simulink model "sim_SMC"  (R2023a)
settings: Solver=VariableStepAuto  StartTime=0.0  StopTime=10.0  RelTol=1e-3
settings Model: Creator=Thu  LastModifiedBy=Thu

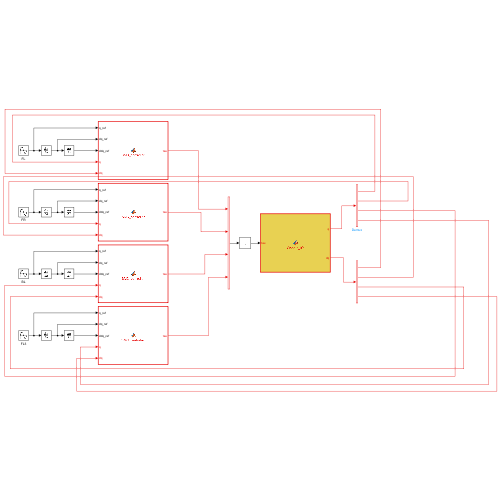
[thumbnail: Simulink's stored preview of the top-level diagram]
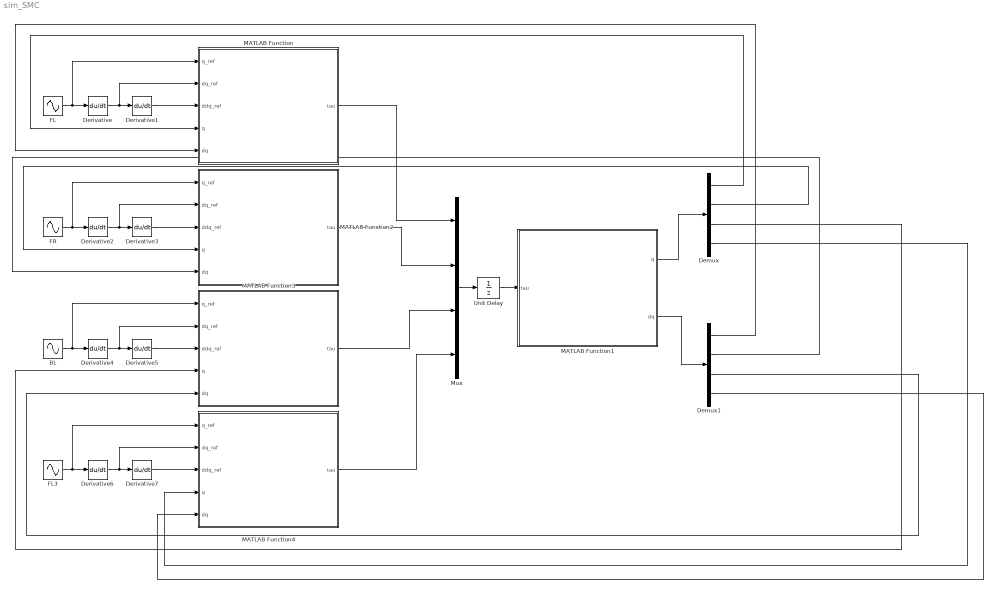
== system sim_SMC ==
  BL : Sin  Amplitude=0.2  Bias=-0.5  SampleTime=0
  Demux : Demux
  Demux1 : Demux
  Derivative{,1..7} (8 alike) : Derivative
  FL : Sin  Amplitude=0.2  Bias=-0.5  SampleTime=0
  FL3 : Sin  Amplitude=0.2  Bias=-0.5  SampleTime=0
  FR : Sin  Amplitude=0.2  Bias=-0.5  SampleTime=0
  MATLAB Function : MATLAB Function  TreatAsAtomicUnit=on
  MATLAB Function1 : MATLAB Function  TreatAsAtomicUnit=on
  MATLAB Function2 : MATLAB Function  TreatAsAtomicUnit=on
  MATLAB Function3 : MATLAB Function  TreatAsAtomicUnit=on
  MATLAB Function4 : MATLAB Function  TreatAsAtomicUnit=on
  Mux : Mux
  Unit Delay : UnitDelay  SampleTime=-1  HasFrameUpgradeWarning=on
  wires:
  FL/1 -> MATLAB Function/1(q_ref), Derivative/1
  Derivative/1 -> MATLAB Function/2(dq_ref), Derivative1/1
  Derivative1/1 -> MATLAB Function/3(ddq_ref)
  Derivative3/1 -> MATLAB Function2/3(ddq_ref)
  Derivative2/1 -> MATLAB Function2/2(dq_ref), Derivative3/1
  FR/1 -> MATLAB Function2/1(q_ref), Derivative2/1
  Derivative5/1 -> MATLAB Function3/3(ddq_ref)
  Derivative4/1 -> MATLAB Function3/2(dq_ref), Derivative5/1
  BL/1 -> MATLAB Function3/1(q_ref), Derivative4/1
  Derivative7/1 -> MATLAB Function4/3(ddq_ref)
  Derivative6/1 -> MATLAB Function4/2(dq_ref), Derivative7/1
  FL3/1 -> MATLAB Function4/1(q_ref), Derivative6/1
  MATLAB Function3/1(tau) -> Mux/3
  MATLAB Function4/1(tau) -> Mux/4
  MATLAB Function2/1(tau) -> Mux/2
  MATLAB Function/1(tau) -> Mux/1
  MATLAB Function1/1(q) -> Demux/1
  MATLAB Function1/2(dq) -> Demux1/1
  Demux/1 -> MATLAB Function/4(q)
  Demux/2 -> MATLAB Function2/4(q)
  Demux/3 -> MATLAB Function3/4(q)
  Demux/4 -> MATLAB Function4/4(q)
  Demux1/1 -> MATLAB Function/5(dq)
  Demux1/2 -> MATLAB Function2/5(dq)
  Demux1/3 -> MATLAB Function3/5(dq)
  Demux1/4 -> MATLAB Function4/5(dq)
  Mux/1 -> Unit Delay/1
  Unit Delay/1 -> MATLAB Function1/1(tau)

== matlab function sim_SMC/MATLAB Function1 ==
  data: tau input; q output; dq output
function [q, dq] = Webots_IO(tau)
    % Khai báo các hàm API từ Webots
    coder.extrinsic('wb_robot_init', 'wb_robot_step', 'wb_motor_set_torque', ...
                    'wb_position_sensor_get_value', 'wb_position_sensor_enable');    
    % Khởi tạo 8 khớp (4 chân x 2 khớp/chân)
    q = zeros(8,1);
    dq = zeros(8,1);
    persistent q_old is_initialized;
    TIME_STEP = 5; 
    
    legs = {'FL', 'FR', 'BL', 'BR'};
    parts = {'hip', 'knee'};
    
    if isempty(is_initialized)
        for i = 1:4
            for j = 1:2
                sensor_name = ['sensor_', legs{i}, '_', parts{j}];
                wb_position_sensor_enable(sensor_name, TIME_STEP);
            end
        end
        q_old = zeros(8,1);
        is_initialized = true;
    end
    
    wb_robot_step(TIME_STEP);
    
    % 2. Gửi Torque (tau) và Đọc góc (q)
    idx = 1;
    for i = 1:4
        for j = 1:2
            motor_name = ['motor_', legs{i}, '_', parts{j}];
            sensor_name = ['sensor_', legs{i}, '_', parts{j}];
            
            % Gửi lực xuống motor
            wb_motor_set_torque(motor_name, tau(idx));
            
            % Đọc góc thực tế (Radian)
            q_raw = wb_position_sensor_get_value(sensor_name);
            
            % Chuẩn hóa 0-360 độ theo logic phần cứng
            q_deg = mod(q_raw * (180/pi), 360);
            q(idx) = q_deg * (pi/180); % Đưa về Radian cho SMC
            
            idx = idx + 1;
        end
    end
    
    % 3. Tính vận tốc dq
    dt = TIME_STEP / 1000;
    dq = (q - q_old) / dt;
    q_old = q;
end

== matlab function sim_SMC/MATLAB Function ==
  data: q_ref input; tau output; dq_ref input; ddq_ref input; q input; dq input
function tau = SMC_controller(q_ref, dq_ref, ddq_ref, q, dq)
    % q_ref, dq_ref, ddq_ref: Quỹ đạo mong muốn [2x1]
    % q, dq: Phản hồi thực tế từ Webots [2x1]
    tau = zeros(2,1);
    
    %% 1. Các thông số bộ điều khiển
    lambda = [15 0; 0 15]; % Ma trận hệ số mặt trượt
    K = [5 0; 0 5];        % Độ lợi điều khiển 
    Phi = [0.1 0; 0 0.1];  % Bề dày lớp biên để chống rung 

    q1 = q(1); q2 = q(2);
    dq1 = dq(1); dq2 = dq(2);

    %% 2. Tính toán Ma trận Động lực học 
    M = [cos(q2)/50 + 0.040128, cos(q2)/100 + 0.0066948;
         cos(q2)/100 + 0.0066948, 0.0066948];
    
    C = [dq2*sin(q2)*(-0.01), sin(q2)*(dq1 + dq2)*(-0.01);
         (dq1*sin(q2))/100, 0];
    
    G = [cos(q1+q2)*0.4905 + cos(q1)*1.962;
         cos(q1+q2)*0.4905];

    %% 3. Thuật toán SMC
    e = q - q_ref;      % Sai số vị trí
    de = dq - dq_ref;   % Sai số vận tốc

    s = de + lambda * e;
    
    % điều khiển tương đương 
    tau_eq = M * (ddq_ref - lambda * de) + C * dq + G;
    
    % điều khiển bù 
    sat_s = saturation_local(s, Phi);
    
    tau_reach = -M * K * sat_s;

    %% 4. Đầu ra mô-men xoắn
    tau = tau_eq + tau_reach;
end

function out = saturation_local(s, Phi)
    out = zeros(2,1);
    for i = 1:2
        if abs(s(i)) > Phi(i,i)
            out(i) = sign(s(i));
        else
            out(i) = s(i) / Phi(i,i);
        end
    end
end

== matlab function sim_SMC/MATLAB Function2 ==
  data: q_ref input; tau output; dq_ref input; ddq_ref input; q input; dq input
function tau = SMC_controller(q_ref, dq_ref, ddq_ref, q, dq)
    % q_ref, dq_ref, ddq_ref: Quỹ đạo mong muốn [2x1]
    % q, dq: Phản hồi thực tế từ Webots [2x1]
    tau = zeros(2,1);
    
    %% 1. Các thông số bộ điều khiển
    lambda = [15 0; 0 15]; % Ma trận hệ số mặt trượt
    K = [5 0; 0 5];        % Độ lợi điều khiển 
    Phi = [0.1 0; 0 0.1];  % Bề dày lớp biên để chống rung 

    q1 = q(1); q2 = q(2);
    dq1 = dq(1); dq2 = dq(2);

    %% 2. Tính toán Ma trận Động lực học 
    M = [cos(q2)/50 + 0.040128, cos(q2)/100 + 0.0066948;
         cos(q2)/100 + 0.0066948, 0.0066948];
    
    C = [dq2*sin(q2)*(-0.01), sin(q2)*(dq1 + dq2)*(-0.01);
         (dq1*sin(q2))/100, 0];
    
    G = [cos(q1+q2)*0.4905 + cos(q1)*1.962;
         cos(q1+q2)*0.4905];

    %% 3. Thuật toán SMC
    e = q - q_ref;      % Sai số vị trí
    de = dq - dq_ref;   % Sai số vận tốc

    s = de + lambda * e;
    
    % điều khiển tương đương 
    tau_eq = M * (ddq_ref - lambda * de) + C * dq + G;
    
    % điều khiển bù 
    sat_s = saturation_local(s, Phi);
    
    tau_reach = -M * K * sat_s;

    %% 4. Đầu ra mô-men xoắn
    tau = tau_eq + tau_reach;
end

function out = saturation_local(s, Phi)
    out = zeros(2,1);
    for i = 1:2
        if abs(s(i)) > Phi(i,i)
            out(i) = sign(s(i));
        else
            out(i) = s(i) / Phi(i,i);
        end
    end
end

== matlab function sim_SMC/MATLAB Function3 ==
  data: q_ref input; tau output; dq_ref input; ddq_ref input; q input; dq input
function tau = SMC_controller(q_ref, dq_ref, ddq_ref, q, dq)
    % q_ref, dq_ref, ddq_ref: Quỹ đạo mong muốn [2x1]
    % q, dq: Phản hồi thực tế từ Webots [2x1]
    tau = zeros(2,1);
    
    %% 1. Các thông số bộ điều khiển 
    lambda = [15 0; 0 15]; % Ma trận hệ số mặt trượt
    K = [5 0; 0 5];        % Độ lợi điều khiển 
    Phi = [0.1 0; 0 0.1];  % Bề dày lớp biên để chống rung 

    q1 = q(1); q2 = q(2);
    dq1 = dq(1); dq2 = dq(2);

    %% 2. Tính toán Ma trận Động lực học 
    M = [cos(q2)/50 + 0.040128, cos(q2)/100 + 0.0066948;
         cos(q2)/100 + 0.0066948, 0.0066948];
    
    C = [dq2*sin(q2)*(-0.01), sin(q2)*(dq1 + dq2)*(-0.01);
         (dq1*sin(q2))/100, 0];
    
    G = [cos(q1+q2)*0.4905 + cos(q1)*1.962;
         cos(q1+q2)*0.4905];

    %% 3. Thuật toán SMC
    e = q - q_ref;      % Sai số vị trí
    de = dq - dq_ref;   % Sai số vận tốc

    s = de + lambda * e;
    
    % điều khiển tương đương 
    tau_eq = M * (ddq_ref - lambda * de) + C * dq + G;
    
    % điều khiển bù 
    sat_s = saturation_local(s, Phi);
    
    tau_reach = -M * K * sat_s;

    %% 4. Đầu ra mô-men xoắn
    tau = tau_eq + tau_reach;
end

function out = saturation_local(s, Phi)
    out = zeros(2,1);
    for i = 1:2
        if abs(s(i)) > Phi(i,i)
            out(i) = sign(s(i));
        else
            out(i) = s(i) / Phi(i,i);
        end
    end
end

== matlab function sim_SMC/MATLAB Function4 ==
  data: q_ref input; tau output; dq_ref input; ddq_ref input; q input; dq input
function tau = SMC_controller(q_ref, dq_ref, ddq_ref, q, dq)
    % q_ref, dq_ref, ddq_ref: Quỹ đạo mong muốn [2x1]
    % q, dq: Phản hồi thực tế từ Webots [2x1]
    tau = zeros(2,1);
    
    %% 1. Các thông số bộ điều khiển 
    lambda = [15 0; 0 15]; % Ma trận hệ số mặt trượt
    K = [5 0; 0 5];        % Độ lợi điều khiển 
    Phi = [0.1 0; 0 0.1];  % Bề dày lớp biên để chống rung 

    q1 = q(1); q2 = q(2);
    dq1 = dq(1); dq2 = dq(2);

    %% 2. Tính toán Ma trận Động lực học 
    M = [cos(q2)/50 + 0.040128, cos(q2)/100 + 0.0066948;
         cos(q2)/100 + 0.0066948, 0.0066948];
    
    C = [dq2*sin(q2)*(-0.01), sin(q2)*(dq1 + dq2)*(-0.01);
         (dq1*sin(q2))/100, 0];
    
    G = [cos(q1+q2)*0.4905 + cos(q1)*1.962;
         cos(q1+q2)*0.4905];

    %% 3. Thuật toán SMC
    e = q - q_ref;      % Sai số vị trí
    de = dq - dq_ref;   % Sai số vận tốc

    s = de + lambda * e;
    
    % điều khiển tương đương 
    tau_eq = M * (ddq_ref - lambda * de) + C * dq + G;
    
    % điều khiển bù 
    sat_s = saturation_local(s, Phi);
    
    tau_reach = -M * K * sat_s;

    %% 4. Đầu ra mô-men xoắn
    tau = tau_eq + tau_reach;
end

function out = saturation_local(s, Phi)
    out = zeros(2,1);
    for i = 1:2
        if abs(s(i)) > Phi(i,i)
            out(i) = sign(s(i));
        else
            out(i) = s(i) / Phi(i,i);
        end
    end
end
